simulink model "Parte2"  (R2021a)
settings: Solver=VariableStepAuto  StartTime=0.0  StopTime=10.0  RelTol=1e-3
undefined symbols (not defined in the file or in its folder): K
settings Model: Creator=josef  LastModifiedBy=josef

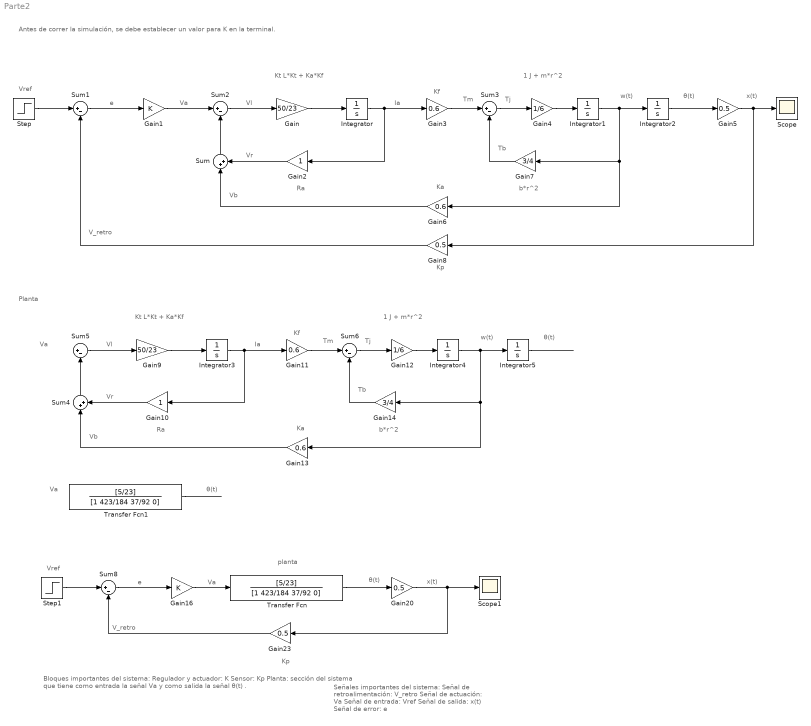
== system Parte2 ==
  note: Vref
  note: e
  note: Va
  note: Vl
  note: Vr
  note: Vb
  note: Kt
      | L*Kt + Ka*Kf
  note: Ia
  note: Ra
  note: Kf
  note: Tm
  note: Tj
  note: 1
      | J + m*r^2
  note: Tb
  note: b*r^2
  note: w(t)
  note: θ(t)
  note: x(t)
  note: V_retro
  note: Ka
  note: Kp
  note: Planta
  note: Antes de correr la simulación, se debe establecer un valor para K en la terminal.
  note: Va
  note: Vl
  note: Vr
  note: Vb
  note: Kt
      | L*Kt + Ka*Kf
  note: Ia
  note: Ra
  note: Kf
  note: Tm
  note: Tj
  note: 1
      | J + m*r^2
  note: Tb
  note: b*r^2
  note: w(t)
  note: θ(t)
  note: Ka
  note: Va
  note: θ(t)
  note: Vref
  note: e
  note: Va
  note: θ(t)
  note: x(t)
  note: V_retro
  note: Kp
  note: planta
  note: Bloques importantes del sistema:
      |
      | Regulador y actuador: K
      | Sensor: Kp
      | Planta: sección del sistema que tiene como entrada la señal Va y como salida la señal θ(t) .
  note: Señales importantes del sistema:
      |
      | Señal de retroalimentación: V_retro
      | Señal de actuación: Va
      | Señal de entrada: Vref
      | Señal de salida: x(t)
      | Señal de error: e
  Gain : Gain  Gain=50/23
  Gain1 : Gain  Gain=K
  Gain10 : Gain
  Gain{3,6,11,13} (4 alike) : Gain  Gain=0.6
  Gain12 : Gain  Gain=1/6
  Gain14 : Gain  Gain=3/4
  Gain16 : Gain  Gain=K
  Gain2 : Gain
  Gain{5,8,20,23} (4 alike) : Gain  Gain=0.5
  Gain4 : Gain  Gain=1/6
  Gain7 : Gain  Gain=3/4
  Gain9 : Gain  Gain=50/23
  Integrator{,1..5} (6 alike) : Integrator
  Scope : Scope
  Scope1 : Scope
  Step : Step  SampleTime=0
  Step1 : Step  SampleTime=0
  Sum : Sum  Inputs=|++
  Sum{1..3,5..6,8} (6 alike) : Sum  Inputs=|+-
  Sum4 : Sum  Inputs=|++
  Transfer Fcn : TransferFcn  Numerator=[5/23]  Denominator=[1 423/184 37/92 0]
  Transfer Fcn1 : TransferFcn  Numerator=[5/23]  Denominator=[1 423/184 37/92 0]
  wires:
  Step/1 -> Sum1/1
  Sum1/1 -> Gain1/1
  Gain1/1 -> Sum2/1
  Sum/1 -> Sum2/2
  Sum2/1 -> Gain/1
  Gain/1 -> Integrator/1
  Gain2/1 -> Sum/2
  Integrator/1 -> Gain3/1, Gain2/1
  Gain3/1 -> Sum3/1
  Sum3/1 -> Gain4/1
  Gain4/1 -> Integrator1/1
  Integrator1/1 -> Gain7/1, Gain6/1, Integrator2/1
  Integrator2/1 -> Gain5/1
  Gain5/1 -> Gain8/1, Scope/1
  Gain6/1 -> Sum/1
  Gain7/1 -> Sum3/2
  Gain8/1 -> Sum1/2
  Gain14/1 -> Sum6/2
  Gain13/1 -> Sum4/1
  Integrator5/1 -> ?
  Integrator4/1 -> Integrator5/1, Gain13/1, Gain14/1
  Gain12/1 -> Integrator4/1
  Sum6/1 -> Gain12/1
  Gain11/1 -> Sum6/1
  Integrator3/1 -> Gain10/1, Gain11/1
  Gain10/1 -> Sum4/2
  Gain9/1 -> Integrator3/1
  Sum5/1 -> Gain9/1
  Sum4/1 -> Sum5/2
  ? -> Sum5/1
  Gain16/1 -> Transfer Fcn/1
  Gain23/1 -> Sum8/2
  Gain20/1 -> Scope1/1, Gain23/1
  Transfer Fcn/1 -> Gain20/1
  Sum8/1 -> Gain16/1
  Step1/1 -> Sum8/1
  Transfer Fcn1/1 -> ?
  ? -> Transfer Fcn1/1
